simulink library "vector_Normalizer_ul"  (R2018b)
settings: Solver=VariableStepAuto  StartTime=0.0  StopTime=10.0  RelTol=1e-3
settings Model: Creator=James Reed  LastModifiedBy=James Reed

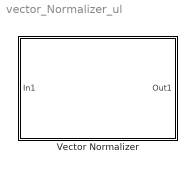
== system vector_Normalizer_ul ==
  "Vector Normalizer " : Subsystem
      mask DialogControl DescTextVar Prompt: %<Vector Normalizer>

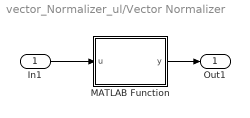
== system vector_Normalizer_ul/Vector Normalizer  ==
  In1 : Inport
  MATLAB Function : MATLAB Function  TreatAsAtomicUnit=on
  Out1 : Outport
  wires:
  MATLAB Function/1(y) -> Out1/1
  In1/1 -> MATLAB Function/1(u)

== matlab function vector_Normalizer_ul/Vector Normalizer /MATLAB Function ==
  data: u input; y output
function y = fcn(u)


 elemNums = numel(u);
 summer = 0;
 for i = 1:elemNums
     
    k = u(i)^2;
    summer = summer + k;
 end 
y = sqrt(summer);
